simulink model "model3"  (R2023a)
settings: Solver=VariableStepAuto  StartTime=0.0  StopTime=5  RelTol=1e-3
values from neighbouring files (symbols this model uses):
  data = load(input_data)    [F1.m]    (also in F1Sy.m; F1Vexp2V.m; F1Vexp2V_SexpS.m; F1Vexp2V_SexpS_ssr.m)
  I = A(3)    [F2.m]    (also in F2P1.m; F2P1_ssr.m = input_parameters(3); F2_ssr.m = input_parameters(3); F3.m)
  J = A(4)    [F3.m]
  R = A(2)    [F1.m]    (also in F1Sy.m; F1Vexp2V.m; F1Vexp2V_SexpS.m; F1Vexp2V_SexpS_ssr_all.m = input_parameters(2))
settings Model: Creator=test  LastModifiedBy=test

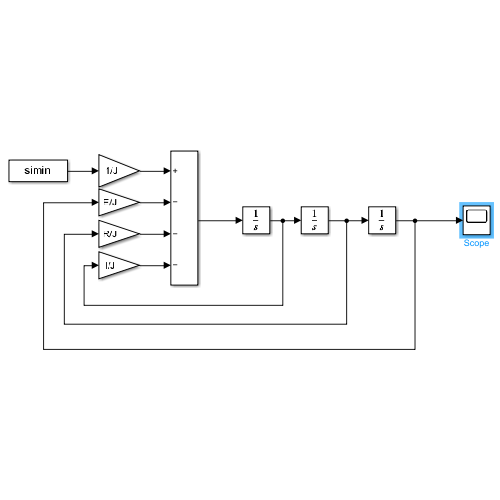
[thumbnail: Simulink's stored preview of the top-level diagram]
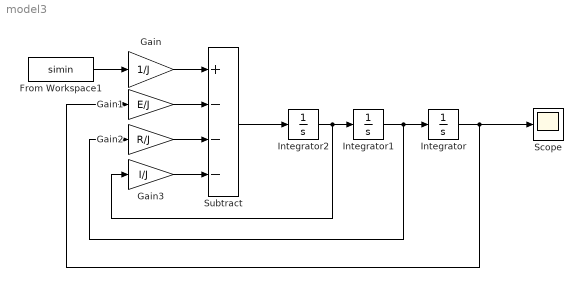
== system model3 ==
  From Workspace1 : FromWorkspace  VariableName=simin
  Gain : Gain  Gain=1/J
  Gain1 : Gain  Gain=E/J
  Gain2 : Gain  Gain=R/J
  Gain3 : Gain  Gain=I/J
  Integrator : Integrator  InitialCondition=data(1,3)
  Integrator1 : Integrator  InitialCondition=data(1,2)
  Integrator2 : Integrator  InitialCondition=data(2,2)-data(1,2)
  Scope : Scope
  Subtract : Sum  Inputs=+---
  wires:
  Integrator1/1 -> Gain2/1, Integrator/1
  Gain1/1 -> Subtract/2
  Gain2/1 -> Subtract/3
  From Workspace1/1 -> Gain/1
  Integrator/1 -> Scope/1, Gain1/1
  Gain/1 -> Subtract/1
  Integrator2/1 -> Gain3/1, Integrator1/1
  Subtract/1 -> Integrator2/1
  Gain3/1 -> Subtract/4
